simulink model "Active_wrist_socket_PROVE_MIE_prova1"  (R2023b)
settings: Solver=ode1  StartTime=0.0  StopTime=inf  FixedStep=0.01  RelTol=1e-3  EnableMultiTasking=on
values from neighbouring files (symbols this model uses):
  dt = 0.005    [model_params.m]
  epsilon_0 = 5    [model_params.m]
  lambda = -2    [model_params.m]
  lambda_feedforward = 0    [model_params.m]
  soglia_nonlin = 0.5    [model_params.m]
undefined symbols (not defined in the file or in its folder): deg, DiscIntNeverNeededParam, m, s
libraries: qbmove_library x4, simulink x3, CP_library x1, QB_pacer_lib x1, SignalEditorBlockLib x1
settings Model: Creator=laurentio  LastModifiedBy=ilari
settings SolverCC: AlgebraicLoopSolver=TrustRegion
settings DataIOCC: LimitDataPoints=on  SaveFormat=Array  ReturnWorkspaceOutputs=off
settings OptimizationCC: LifeSpan=inf
settings DebuggingCC: UnderspecifiedInitializationDetection=Classic  MergeDetectMultiDrivingBlocksExec=none  SolverPrmCheckMsg=warning  UnconnectedInputMsg=warning  UnconnectedOutputMsg=warning  UnconnectedLineMsg=warning  AllowSymbolicDim=off  StateNameClashWarn=warning  SFUnexpectedBacktrackingDiag=warning  SFNoUnconditionalDefaultTransitionDiag=warning  SFExecutionAtInitializationDiag=none  ArithmeticOperatorsInVariantConditions=warning
settings HardwareCC: ProdBitPerPointer=32  ProdBitPerSizeT=32  ProdBitPerPtrDiffT=32  ProdLargestAtomicFloat=None  ProdIntDivRoundTo=Undefined  ProdEndianess=Unspecified  ProdWordSize=32  ProdHWDeviceType=32-bit Generic
settings ModelReferenceCC: EnableRefExpFcnMdlSchedulingChecks=on  PropagateSignalLabelsOutOfModel=off
settings SFSimCC: SimUseLocalCustomCode=off  CustomCodeUndefinedFunction=UseInterfaceOnly
settings RTWCC: RTWUseLocalCustomCode=off
settings CodeAppCC: StateflowObjectComments=on
settings GRTTargetCC: TargetLangStandard=C89/C90 (ANSI)
settings ConfigComp: CovMetricSettings=dw  CovSaveCumulativeToWorkspaceVar=on  CovSaveSingleToWorkspaceVar=on  CovExternalEMLEnable=off  CovSFcnEnable=off

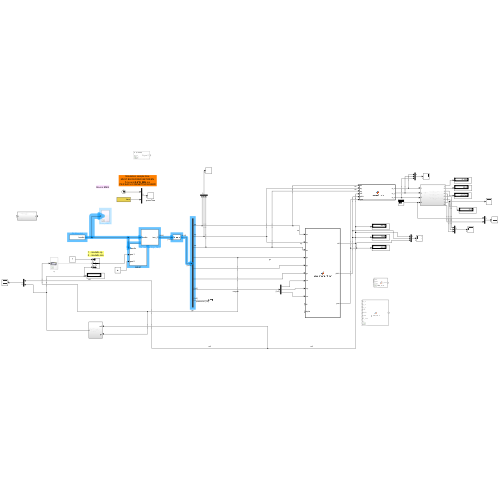
[thumbnail: Simulink's stored preview of the top-level diagram]
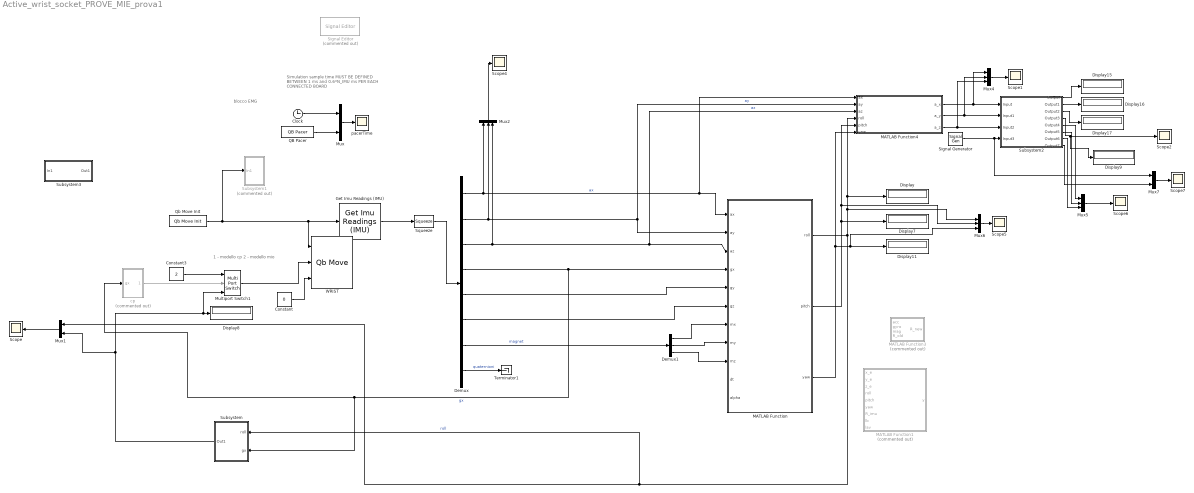
== system Active_wrist_socket_PROVE_MIE_prova1 ==
  note: blocco EMG
  note: 1 - modello cp
      | 2 - modello mio
  note: Simulation sample time
      | MUST BE DEFINED BETWEEN
      | 1 ms and 0.6*N_IMU ms
      | PER EACH CONNECTED BOARD
  Clock : Clock
  Constant : Constant  Value=0
  Constant3 : Constant  Value=2
  Demux : Demux  Outputs=[1 1 1 1 1 1 3 5]
  Demux1 : Demux  Outputs=3
  Display{,7..9,11,15..17} (8 alike) : Display
  Get Imu Readings (IMU) : CP_library/Get Imu Readings (IMU)  ID=2  N_IMU=1  DAISY_CHAINING=off  ACC_UNITY=m/(s^2)  GYRO_UNITY=deg/s  MAG_UNITY=uT
      settings: SourceProductName=Centro Piaggio Library
  MATLAB Function : MATLAB Function  TreatAsAtomicUnit=on
  MATLAB Function1 : MATLAB Function  Commented=on  TreatAsAtomicUnit=on
  MATLAB Function3 : MATLAB Function  Commented=on  TreatAsAtomicUnit=on
  MATLAB Function4 : MATLAB Function  TreatAsAtomicUnit=on
  Multiport Switch1 : MultiPortSwitch  Inputs=2  SaturateOnIntegerOverflow=off  InputSameDT=off
  Mux : Mux  Inputs=2
  Mux1 : Mux  Inputs=2
  Mux{2,4..6} (4 alike) : Mux  Inputs=3
  Mux7 : Mux  Inputs=2
  QB Pacer : QB_pacer_lib/QB Pacer  simTimePerRealTime=1
      settings: SourceProductName=QB Pacer
  Qb Move Init : qbmove_library/Qb Move Init  NUMBER_OF_COM='COM9'  BAUD_RATE_COM=2000000
      settings: SourceProductName=Qb Move Library
  Scope{,1..2,4..7} (7 alike) : Scope
  Signal Generator : SignalGenerator
  Signal Editor : SignalEditorBlockLib/Signal Editor  Commented=on  FileName=signal_generator_piecewise.mat  ActiveScenario=Scenario  ActiveSignal=Signal 1  IsBus=off  OutputBusObjectStr=Bus: BusObject  SampleTime=0  Interpolate=off  ZeroCross=off  OutputAfterFinalValue=Setting to zero  Unit=inherit  PreserveSignalName=on  ApplySigPropsToAllScenarios=on  ApplySigPropsToAllSignals=off
  Squeeze : Squeeze
  Subsystem : Subsystem
  Subsystem1 : Subsystem  Commented=on
  Subsystem2 : Subsystem
  Subsystem3 : Subsystem
  Terminator1 : Terminator
  WRIST : qbmove_library/Qb Move  ID=2  ACTIVE_COMM_DIRECTIONS=Tx  CONTROL_MODE=Prime Movers Positions  DAISY_CHAINING=off  MAX_ANG=0  SW_LIMIT=inf  OFFSET=0  ACTIVATE=on  WDT=0.0  UNIT=TICK
      settings: SourceProductName=Qb Move Library
  cp : Subsystem  Commented=on
  pacerTime : Scope
  wires:
  QB Pacer/1 -> Mux/2
  Clock/1 -> Mux/1
  Mux/1 -> pacerTime/1
  Get Imu Readings (IMU)/1 -> Squeeze/1
  Constant/1 -> WRIST/3
  Squeeze/1 -> Demux/1
  Demux/1 -> Mux2/1, MATLAB Function4/1(ax), MATLAB Function/1(ax)  "ax"
  Demux/2 -> MATLAB Function4/2(ay), MATLAB Function/2(ay), Mux2/2  "ay"
  Demux/3 -> MATLAB Function/3(az), MATLAB Function4/3(az), Mux2/3  "az"
  Demux/4 -> MATLAB Function/4(gx), Subsystem/2(gx), cp/1(gx)  "gx"
  Qb Move Init/1 -> Get Imu Readings (IMU)/1, WRIST/1, Subsystem1/1(In1)
  Constant3/1 -> Multiport Switch1/1
  cp/1(Out1) -> Multiport Switch1/2
  MATLAB Function/1(roll) -> Subsystem/1(roll), Mux1/1, MATLAB Function4/4(roll), Display/1, Mux6/1  "roll"
  MATLAB Function/2(pitch) -> MATLAB Function4/5(pitch), Mux6/2, Display7/1
  MATLAB Function/3(yaw) -> MATLAB Function4/6(yaw), Mux6/3, Display11/1
  Mux1/1 -> Scope/1
  Multiport Switch1/1 -> WRIST/2
  Subsystem/1(Out1) -> Mux1/2, Multiport Switch1/3, Display8/1
  Demux/7 -> Demux1/1  "magnet"
  Demux/8 -> Terminator1/1  "quaternioni"
  Mux2/1 -> Scope4/1
  Subsystem2/1(Output) -> Display15/1
  Subsystem2/2(Output1) -> Display16/1
  Subsystem2/3(Output2) -> Display17/1
  Mux4/1 -> Scope1/1
  MATLAB Function4/1(a_x) -> Mux4/1, Subsystem2/1(Input)
  Mux6/1 -> Scope5/1
  Subsystem2/4(Output3) -> Display9/1, Scope2/1
  MATLAB Function4/2(a_y) -> Mux4/2, Subsystem2/2(Input1)
  MATLAB Function4/3(a_z) -> Mux4/3, Subsystem2/3(Input2)
  Subsystem2/5(Output4) -> Mux5/1
  Subsystem2/6(Output5) -> Mux5/2
  Subsystem2/7(Output6) -> Mux5/3
  Mux5/1 -> Scope6/1
  Signal Generator/1 -> Mux7/1, Subsystem2/4(Input3)
  Mux7/1 -> Scope7/1
  Subsystem2/8(Output7) -> Mux7/2
  Demux/5 -> MATLAB Function/5(gy)
  Demux/6 -> MATLAB Function/6(gz)
  Demux1/1 -> MATLAB Function/7(mx)
  Demux1/2 -> MATLAB Function/8(my)
  Demux1/3 -> MATLAB Function/9(mz)

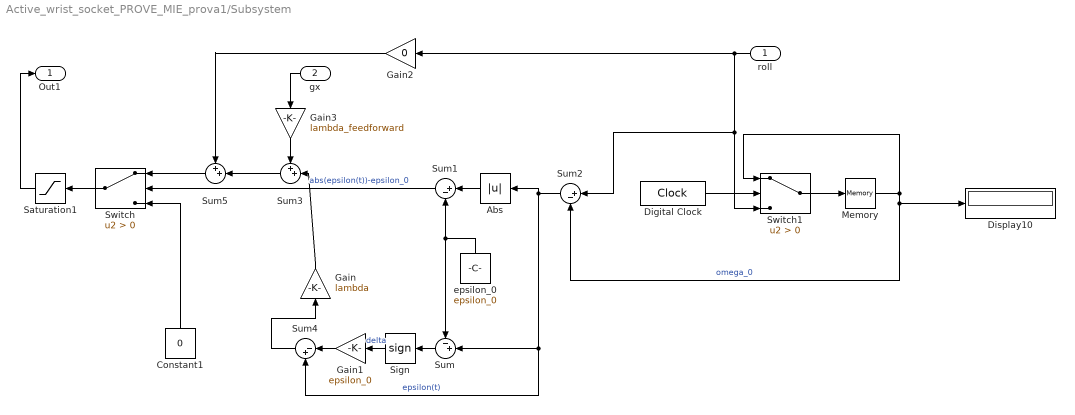
== system Active_wrist_socket_PROVE_MIE_prova1/Subsystem ==
  roll : Inport
  gx : Inport  Port=2
  Abs : Abs  SaturateOnIntegerOverflow=off
  Constant1 : Constant  Value=0
  Digital Clock : DigitalClock  SampleTime=dt
  Display10 : Display
  Gain : Gain  Gain=lambda
  Gain1 : Gain  Gain=epsilon_0
  Gain2 : Gain  Gain=0
  Gain3 : Gain  Gain=lambda_feedforward
  Memory : Memory
  Saturation1 : Saturate  UpperLimit=100  LowerLimit=-100
  Sign : Signum
  Sum : Sum  Inputs=-+|
  Sum1 : Sum  Inputs=|+-
  Sum2 : Sum  Inputs=|+-
  Sum3 : Sum  Inputs=++|
  Sum4 : Sum  Inputs=|-+
  Sum5 : Sum  Inputs=++|
  Switch : Switch  Criteria=u2 > Threshold  SaturateOnIntegerOverflow=off  InputSameDT=off
  Switch1 : Switch  Criteria=u2 > Threshold  SaturateOnIntegerOverflow=off  InputSameDT=off
  epsilon_0 : Constant  Value=epsilon_0
  Out1 : Outport
  wires:
  Gain/1 -> Sum3/2
  Switch/1 -> Saturation1/1
  Sum2/1 -> Abs/1, Sum/2, Sum4/2  "epsilon(t)"
  Sign/1 -> Gain1/1  "delta"
  epsilon_0/1 -> Sum/1, Sum1/2
  roll/1 -> Switch1/3, Sum2/1, Gain2/1
  Switch1/1 -> Memory/1
  Sum4/1 -> Gain/1
  Abs/1 -> Sum1/1
  Sum/1 -> Sign/1
  Constant1/1 -> Switch/3
  Digital Clock/1 -> Switch1/2
  Sum1/1 -> Switch/2  "abs(epsilon(t))-epsilon_0"
  Gain1/1 -> Sum4/1
  Memory/1 -> Sum2/2, Display10/1, Switch1/1  "omega_0"
  Gain3/1 -> Sum3/1
  gx/1 -> Gain3/1
  Saturation1/1 -> Out1/1
  Sum3/1 -> Sum5/2
  Sum5/1 -> Switch/1
  Gain2/1 -> Sum5/1

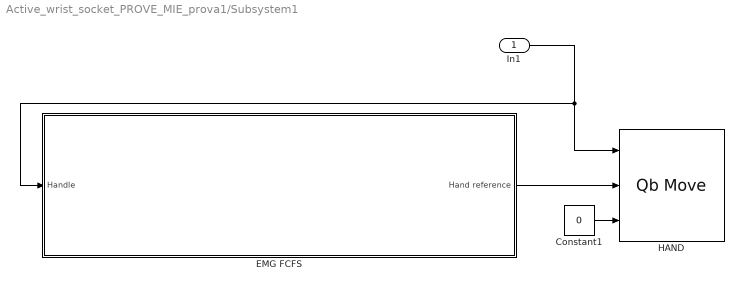
== system Active_wrist_socket_PROVE_MIE_prova1/Subsystem1 ==
  In1 : Inport
  Constant1 : Constant  Value=0
  EMG FCFS : Subsystem
  HAND : qbmove_library/Qb Move  ID=1  ACTIVE_COMM_DIRECTIONS=Tx  CONTROL_MODE=Prime Movers Positions  DAISY_CHAINING=off  MAX_ANG=0  SW_LIMIT=inf  OFFSET=0  ACTIVATE=on  WDT=0.0  UNIT=TICK
      settings: SourceProductName=Qb Move Library
  wires:
  In1/1 -> HAND/1, EMG FCFS/1(Handle)
  Constant1/1 -> HAND/3
  EMG FCFS/1(Hand reference) -> HAND/2

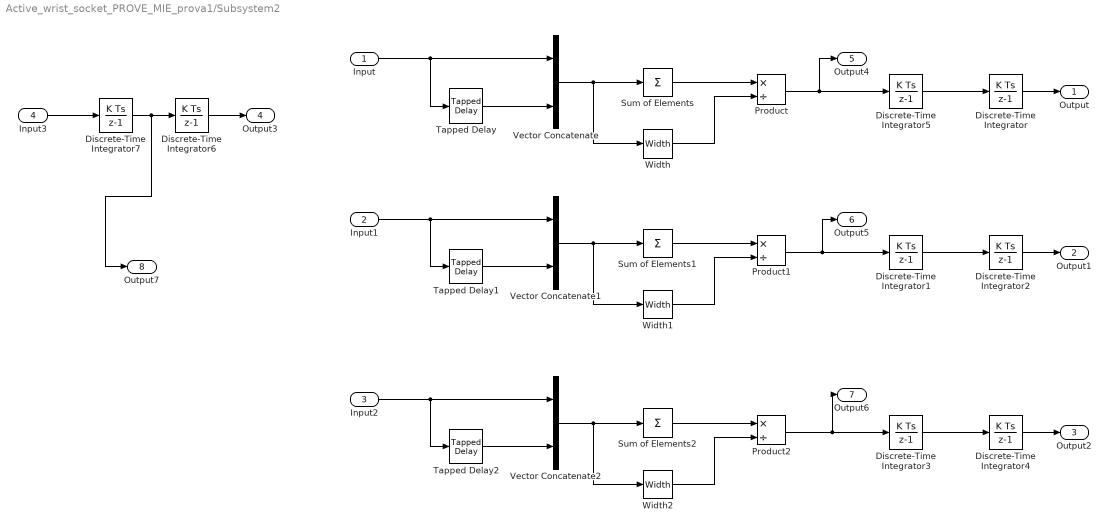
== system Active_wrist_socket_PROVE_MIE_prova1/Subsystem2 ==
  Input : Inport
  Input1 : Inport  Port=2
  Input2 : Inport  Port=3
  Input3 : Inport  Port=4
  Discrete-Time Integrator{,1..7} (8 alike) : DiscreteIntegrator  SampleTime=-1  ICPrevOutput=DiscIntNeverNeededParam  ICPrevScaledInput=DiscIntNeverNeededParam
  Product : Product  Inputs=*/
  Product1 : Product  Inputs=*/
  Product2 : Product  Inputs=*/
  Sum of Elements : Sum  Inputs=+
  Sum of Elements1 : Sum  Inputs=+
  Sum of Elements2 : Sum  Inputs=+
  Tapped Delay : simulink/Discrete/Tapped Delay  vinit=0.0  samptime=-1  NumDelays=31  DelayOrder=Oldest  includeCurrent=off
  Tapped Delay1 : simulink/Discrete/Tapped Delay  vinit=0.0  samptime=-1  NumDelays=31  DelayOrder=Oldest  includeCurrent=off
  Tapped Delay2 : simulink/Discrete/Tapped Delay  vinit=0.0  samptime=-1  NumDelays=31  DelayOrder=Oldest  includeCurrent=off
  Vector Concatenate : Concatenate
  Vector Concatenate1 : Concatenate
  Vector Concatenate2 : Concatenate
  Width : Width
  Width1 : Width
  Width2 : Width
  Output : Outport
  Output1 : Outport  Port=2
  Output2 : Outport  Port=3
  Output3 : Outport  Port=4
  Output4 : Outport  Port=5
  Output5 : Outport  Port=6
  Output6 : Outport  Port=7
  Output7 : Outport  Port=8
  wires:
  Input/1 -> Tapped Delay/1, Vector Concatenate/1
  Tapped Delay/1 -> Vector Concatenate/2
  Vector Concatenate/1 -> Width/1, Sum of Elements/1
  Sum of Elements/1 -> Product/1
  Width/1 -> Product/2
  Product/1 -> Output4/1, Discrete-Time Integrator5/1
  Tapped Delay1/1 -> Vector Concatenate1/2
  Vector Concatenate1/1 -> Width1/1, Sum of Elements1/1
  Product1/1 -> Output5/1, Discrete-Time Integrator1/1
  Width1/1 -> Product1/2
  Input1/1 -> Tapped Delay1/1, Vector Concatenate1/1
  Sum of Elements1/1 -> Product1/1
  Tapped Delay2/1 -> Vector Concatenate2/2
  Vector Concatenate2/1 -> Width2/1, Sum of Elements2/1
  Product2/1 -> Output6/1, Discrete-Time Integrator3/1
  Width2/1 -> Product2/2
  Input2/1 -> Tapped Delay2/1, Vector Concatenate2/1
  Sum of Elements2/1 -> Product2/1
  Discrete-Time Integrator5/1 -> Discrete-Time Integrator/1
  Discrete-Time Integrator1/1 -> Discrete-Time Integrator2/1
  Discrete-Time Integrator3/1 -> Discrete-Time Integrator4/1
  Discrete-Time Integrator/1 -> Output/1
  Discrete-Time Integrator2/1 -> Output1/1
  Discrete-Time Integrator4/1 -> Output2/1
  Discrete-Time Integrator6/1 -> Output3/1
  Discrete-Time Integrator7/1 -> Output7/1, Discrete-Time Integrator6/1
  Input3/1 -> Discrete-Time Integrator7/1

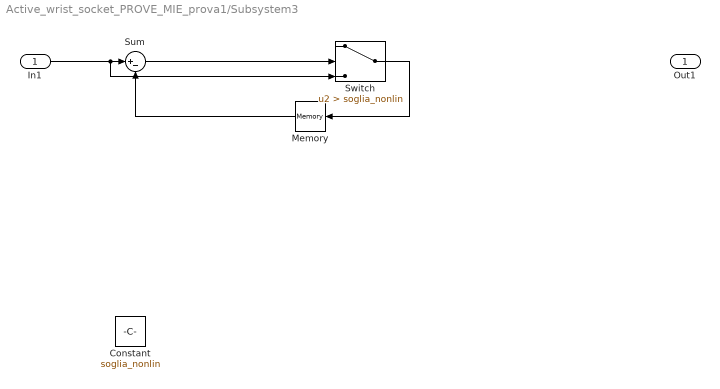
== system Active_wrist_socket_PROVE_MIE_prova1/Subsystem3 ==
  In1 : Inport
  Constant : Constant  Value=soglia_nonlin
  Memory : Memory
  Sum : Sum  Inputs=|+-
  Switch : Switch  Criteria=u2 > Threshold  Threshold=soglia_nonlin  SaturateOnIntegerOverflow=off  InputSameDT=off
  Out1 : Outport
  wires:
  In1/1 -> Switch/3, Sum/1
  Sum/1 -> Switch/2
  Switch/1 -> Memory/1
  Memory/1 -> Sum/2

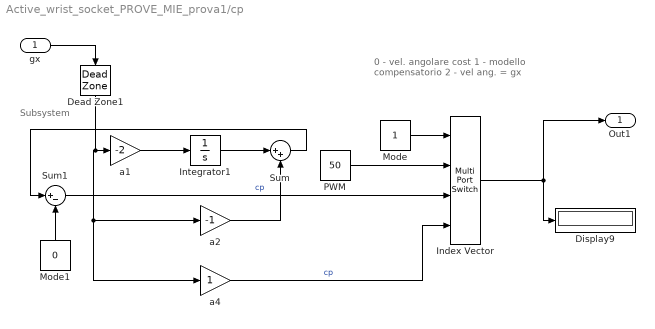
== system Active_wrist_socket_PROVE_MIE_prova1/cp ==
  note: Subsystem
  note: 0 - vel. angolare cost
      | 1 - modello compensatorio
      | 2 - vel ang. = gx
  gx : Inport
  Dead Zone1 : DeadZone  LowerValue=-5  UpperValue=5  LinearizeAsGain=off
  Display9 : Display
  Index Vector : MultiPortSwitch  DataPortOrder=Zero-based contiguous  zeroidx=on  SaturateOnIntegerOverflow=off  InputSameDT=off
  Integrator1 : Integrator
  Mode : Constant
  Mode1 : Constant  Value=0
  PWM : Constant  Value=50
  Sum : Sum  Inputs=|++
  Sum1 : Sum  Inputs=|+-
  a1 : Gain  Gain=-2
  a2 : Gain  Gain=-1
  a4 : Gain
  Out1 : Outport
  wires:
  gx/1 -> Dead Zone1/1
  Index Vector/1 -> Out1/1, Display9/1
  Mode/1 -> Index Vector/1
  a1/1 -> Integrator1/1
  Sum1/1 -> Index Vector/3  "cp"
  PWM/1 -> Index Vector/2
  a4/1 -> Index Vector/4  "cp"
  a2/1 -> Sum/2
  Sum/1 -> Sum1/1
  Mode1/1 -> Sum1/2
  Integrator1/1 -> Sum/1
  Dead Zone1/1 -> a2/1, a4/1, a1/1

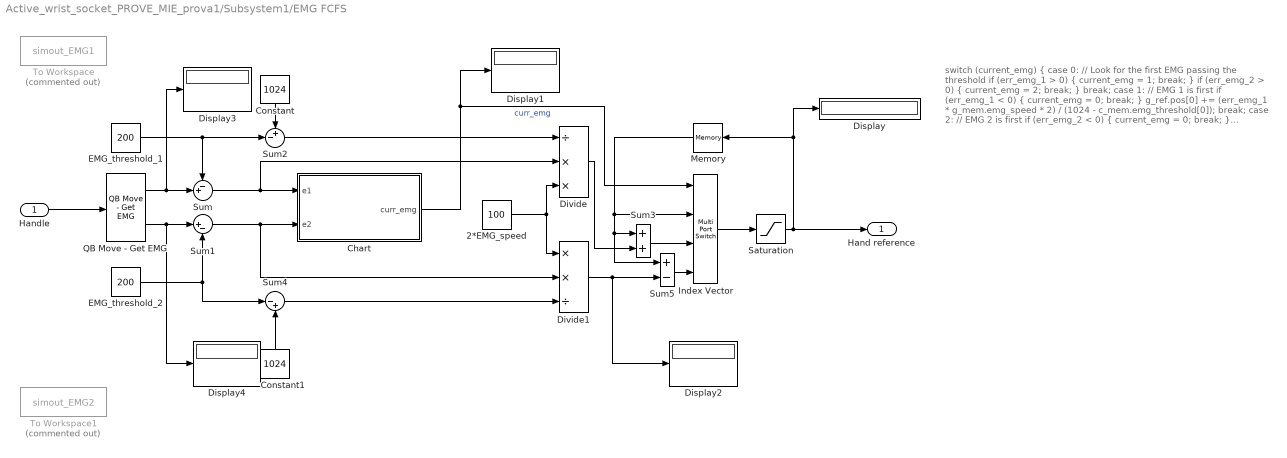
== system Active_wrist_socket_PROVE_MIE_prova1/Subsystem1/EMG FCFS ==
  note: switch (current_emg) {
      | case 0:
      | // Look for the first EMG passing the threshold
      | if (err_emg_1 > 0) {
      | current_emg = 1;
      | break;
      | }
      | if (err_emg_2 > 0) {
      | current_emg = 2;
      | break;
      | }
      | break;
      |
      | case 1:
      | // EMG 1 is first
      | if (err_emg_1 < 0) {
      | current_emg = 0;
      | break;
      | }
      | g_ref.pos[0] += (err_emg_1 * g_mem.emg_speed * 2) / (1024 - c_mem.emg_threshold[0]);
      | break;
      |
      | case 2:
      | // EMG 2 is first
      | if (err_emg_2 < 0) {
      | current_emg = 0;
      | break;
      | }
      | g_ref.pos[0] -= (err_emg_2 * g_mem.emg_speed * 2) / (1024 - c_mem.emg_threshold[1]);
      | break;
      |
      | default:
      | break;
      | }
  Handle : Inport
  2*EMG_speed : Constant  Value=100
  Chart : Stateflow chart  TreatAsAtomicUnit=on
  Constant : Constant  Value=1024
  Constant1 : Constant  Value=1024
  Display{,1..4} (5 alike) : Display
      Display settings: Format=decimal (Stored Integer)
  Divide : Product  Inputs=/**
  Divide1 : Product  Inputs=**/
  EMG_threshold_1 : Constant  Value=200
  EMG_threshold_2 : Constant  Value=200
  Index Vector : MultiPortSwitch  DataPortOrder=Zero-based contiguous  zeroidx=on  SaturateOnIntegerOverflow=off  InputSameDT=off
  Memory : Memory
  QB Move - Get EMG : qbmove_library/QB Move - Get EMG  ID=2  DAISY_CHAINING=off
      settings: SourceProductName=Qb Move Library
  Saturation : Saturate  UpperLimit=19000  LowerLimit=0
  Sum : Sum  Inputs=-+|
  Sum1 : Sum  Inputs=|+-
  Sum2 : Sum  Inputs=+-|
  Sum3 : Sum
  Sum4 : Sum  Inputs=|-+
  Sum5 : Sum  Inputs=+-
  To Workspace : ToWorkspace  Commented=on  VariableName=simout_EMG1  SaveFormat=Timeseries  SampleTime=-1
  To Workspace1 : ToWorkspace  Commented=on  VariableName=simout_EMG2  SaveFormat=Timeseries  SampleTime=-1
  Hand reference : Outport
  wires:
  Memory/1 -> Index Vector/2, Sum5/1, Sum3/1
  Sum5/1 -> Index Vector/4
  Sum1/1 -> Divide1/2, Chart/2(e2)
  2*EMG_speed/1 -> Divide1/1, Divide/3
  Constant1/1 -> Sum4/2
  Chart/1(curr_emg) -> Display1/1, Index Vector/1  "curr_emg"
  Sum3/1 -> Index Vector/3
  Sum/1 -> Divide/2, Chart/1(e1)
  Index Vector/1 -> Saturation/1
  QB Move - Get EMG/1 -> Display3/1, Sum/2
  Sum4/1 -> Divide1/3
  Divide/1 -> Sum3/2
  Constant/1 -> Sum2/1
  EMG_threshold_1/1 -> Sum2/2, Sum/1
  Divide1/1 -> Display2/1, Sum5/2
  Handle/1 -> QB Move - Get EMG/1
  QB Move - Get EMG/2 -> Display4/1, Sum1/1
  Sum2/1 -> Divide/1
  Saturation/1 -> Hand reference/1, Display/1, Memory/1
  EMG_threshold_2/1 -> Sum4/1, Sum1/2

== matlab function Active_wrist_socket_PROVE_MIE_prova1/MATLAB Function1 ==
  data: x_e input; y_e input; z_e input; roll input; y output; pitch input; yaw input; R_imu input; lb input; lav input
function y = jacobians(x_e , y_e , z_e ,roll, pitch, yaw, R_imu, lb , lav)


rotation_matrix

J1= [0;
    -lb*cosd(theta3)-lav*cosd(theta3+theta6);
    lb*cosd(theta2)+lav*cosd(theta2+theta5);
    1;
    0;
    0];

J2= [lb*cosd(theta3)+lav*cosd(theta3+theta6);
    0;
    -lb*cosd(theta1)-lav*cosd(theta1+theta4);
    0;
    1;
    0];

J3 = [-lb*cosd(theta2)-lav*cosd(theta2+theta5);
      lb*cosd(theta1)+lav*cosd(theta1+theta4);
      0;
      0;
      0;
      1];

J4= [0;
    -lav*cosd(theta3+theta6);
    lav*cosd(theta2+theta5);
    1;
    0;
    0];


J5= [lav*cosd(theta3+theta6);
    0;
    -lav*cosd(theta1+theta4);
    0;
    1;
    0];

J6 = [-lav*cosd(theta2+theta5);
      lav*cosd(theta1+theta4);
      0;
      0;
      0;
      1];

Jtot = [J1 J2 J3 J4 J5 J6];

x = [x_e ; y_e ; z_e ; roll ; pitch ; yaw]; %ingresso

== matlab function Active_wrist_socket_PROVE_MIE_prova1/MATLAB Function ==
  settings: updateMethod=DISCRETE
  data: ax input; roll output; ay input; az input; gx input; gy input; gz input; mx input; my input; mz input; dt input; pitch output; yaw output; alpha input
% function [roll, pitch, yaw] = fusione(ax, ay, az, gx, gy, gz, mx, my, mz, dt, alpha)
% 
% 
% accelReadings = [ax , ay , az];
% gyroReadings = [gx , gy , gz];
% magReadings = [mx , my , mz];
% 
% 
% fuse = complementaryFilter;
% 
% [orientation,angularVelocity] = fuse(accelReadings,gyroReadings,magReadings
% 
% eul = quat2eul(orientation)
% 
% roll = eul(1);
% pitch = eul(2);
% yaw = eul(3);

% versione uno
function [roll, pitch, yaw] = complementaryFilter(ax, ay, az, gx, gy, gz, mx, my, mz, dt, alpha)
    % ax, ay, az: dati dell'accelerometro
    % gx, gy, gz: dati del giroscopio (in gradi al secondo)
    % mx, my, mz: dati del magnetometro
    % dt: passo di campionamento
    % alpha: coefficiente del filtro

    persistent roll_prev pitch_prev yaw_prev;

    if isempty(roll_prev)
        roll_prev = 0;
        pitch_prev = 0;
        yaw_prev = 0;
    end

    % Calcola roll e pitch dall'accelerometro in gradi
    roll_acc = atan2d(ay, az);
    pitch_acc = atan2d(-ax, sqrt(ay^2 + az^2));
    % pitch_acc = atan2d(-ax, az);


    %  % Correzione della gamma per il pitch 
    % if az < 0
    %     if pitch_acc > 0
    %         pitch_acc = 180 - pitch_acc;
    %     else
    %         pitch_acc = -180 - pitch_acc;
    %     end
    % end
    % 


    % Calcola yaw dal magnetometro in gradi
    % Compensa il roll e pitch utilizzando i dati dell'accelerometro
    mag_x_comp = mx * cosd(pitch_acc) + my * sind(roll_acc) * sind(pitch_acc) + mz * cosd(roll_acc) * sind(pitch_acc);
    mag_y_comp = my * cosd(roll_acc) - mz * sind(roll_acc);
    yaw_mag = atan2d(-mag_y_comp, mag_x_comp);

    % Integra i dati del giroscopio per ottenere roll, pitch e yaw in gradi
    roll_gyro = gx * dt;
    pitch_gyro = gy * dt;
    yaw_gyro = gz * dt;

    % Somma cumulativa degli angoli integrati
    roll_gyro_total = roll_prev + roll_gyro;
    pitch_gyro_total = pitch_prev + pitch_gyro;
    yaw_gyro_total = yaw_prev + yaw_gyro;

    % Applica il filtro complementare
    roll = alpha * roll_gyro_total + (1 - alpha) * roll_acc;
    pitch = alpha * pitch_gyro_total + (1 - alpha) * pitch_acc;
    yaw = alpha * yaw_gyro_total + (1 - alpha) * yaw_mag;

    % % roll = roll + 180;
    % % pitch = pitch + 180;
    % % yaw = yaw + 180;


 % % Correzione degli angoli per mantenere gli intervalli appropriati
 %    if roll > pi
 %        roll = roll - 2*pi;
 %    elseif roll < -pi
 %        roll = roll + 2*pi;
 %    end
 % 
 %    if pitch > pi
 %        pitch = pitch - 2*pi;
 %    elseif pitch < -pi
 %        pitch = pitch + 2*pi;
 %    end
 % 
 %    if yaw > pi
 %        yaw = yaw - 2*pi;
 %    elseif yaw < -pi
 %        yaw = yaw + 2*pi;
 %    end

    % Aggiorna gli angoli precedenti
    roll_prev = roll;
    pitch_prev = pitch;
    yaw_prev = yaw;
end

%% versione due

% 
%  VERSIONE VECCHIA 
%     ax, ay, az: accelerometer data
%     gx, gy, gz: gyroscope data
%     dt: time step
%     alpha: filter coefficient
% 
% 
%     persistent roll_pre pitch_pre yaw_pre;
% 
%     if isempty(roll_pre)
%         roll_pre = 0;
%         pitch_pre = 0;
%         yaw_pre= 0;
%     end
% 
%     % Calcola roll e pitch dall'accelerometro in gradi
%     roll_acc = atan2(ay, az) * (180/pi);
%     pitch_acc = atan2(-ax, sqrt(ay^2 + az^2)) * (180/pi);
% 
%     % Integra i dati del giroscopio per ottenere roll, pitch e yaw
%     roll_gyro = gx * dt;
%     pitch_gyro = gy * dt;
%     yaw_gyro = gz * dt;
% 
%     % Applica il filtro complementare
%     roll = (alpha * (roll_pre + roll_gyro) + (1 - alpha) * roll_acc) ;
%     pitch = (alpha * (pitch_pre + pitch_gyro) + (1 - alpha) * pitch_acc) ;
%     yaw = yaw_pre + yaw_gyro ;  % Senza magnetometro, usiamo solo il giroscopio
% 
%     % Aggiorna gli angoli precedenti
%     roll_pre = roll;
%     pitch_pre = pitch;
%     yaw_pre = yaw;
% 
% 
% 
% end

== stateflow chart Active_wrist_socket_PROVE_MIE_prova1/Subsystem1/EMG FCFS/Chart ==
  state State0
    entry: curr_emg = 0;
  state State1
    entry: curr_emg = 1;
  state State2
    entry: curr_emg = 2;
  (default) -> State0
  State0 -> State1 [order 1] : [e1 > 0]
  State1 -> State0 : [e1 < 0]
  State2 -> State0 : [e2 < 0]
  State0 -> State2 [order 2] : [e2 > 0]
  data: e1 input; e2 input; curr_emg output

== matlab function Active_wrist_socket_PROVE_MIE_prova1/MATLAB Function4 ==
  data: ax input; ay input; az input; a_x output; roll input; pitch input; yaw input; a_y output; a_z output
function [a_x, a_y, a_z ] = removeGravity(ax, ay, az, roll, pitch, yaw)
    gravity = [0; 0; 9.81]; % 3x1
    acc= [ax ay az]; %1x3
   % 
   % roll = roll + 180;
   % pitch = pitch +180;
   % yaw = yaw + 180;
   % 

    Rx = [1, 0, 0;
          0, cosd(roll), -sind(roll);
          0, sind(roll), cosd(roll)];
      
    Ry = [cosd(pitch), 0, sind(pitch);
          0, 1, 0;
          -sind(pitch), 0, cosd(pitch)];
      
    Rz = [cosd(yaw), -sind(yaw), 0;
          sind(yaw), cosd(yaw), 0;
          0, 0, 1];
      
    R = Rz * Ry * Rx;

    % Converti gli angoli di Eulero in matrice di rotazione
    rotation_matrix = R';
    correction = rotation_matrix * gravity; %3x1


    % Sottrai la gravità
    acc_corrected = acc - correction'; %1x3
    a_x = acc_corrected(1); 
    a_y = acc_corrected(2);
    a_z = acc_corrected(3);

end

== matlab function Active_wrist_socket_PROVE_MIE_prova1/MATLAB Function3 ==
  data: R_new output; acc input; gyro input; mag input; R_old input
function R_new = mh_filter(acc, gyro, mag, R_old)

ax = acc(1);
ay = acc(2);
az = acc(3);

gx = gyro(1);
gy = gyro(2);
gz = gyro(3);

mx = mag(1);
my = mag(2);
my = mag(3);

% normalizzo vettori di campo magnetico e gravitazionale

abn = acc(1 , :)./abs(acc(1 , :));
mbn = mag(1 , :)./abs(mag(1 , :));


%considero un reference frame classico , levogiro con z verso l'alto
%calcolo  vettore gravità nel frame body
